simulink model "dblpend1"  (Simulink 6.0)
settings: Solver=ode45  SolverMode=SingleTasking  StartTime=0  StopTime=10000  MaxStep=0.05  RelTol=1e-5  AbsTol=1e-6
PreLoadFcn:
  | l21=5;w21=5;n1=1/4;e1=1/2;
settings Model: Creator=The MathWorks Inc.  LastModifiedBy=batserve  ExtModeTrigMode=oneshot  ExtModeAutoUpdateStatusClock=off
settings DataIOCC: InitialState=xFinal  LimitDataPoints=off  SaveOutput=off  SaveTime=off
settings OptimizationCC: BooleanDataType=off
settings DebuggingCC: CheckExecutionContextPreStartOutputMsg=on  CheckExecutionContextRuntimeOutputMsg=on  SolverPrmCheckMsg=none
settings HardwareCC: TargetUnknown=on

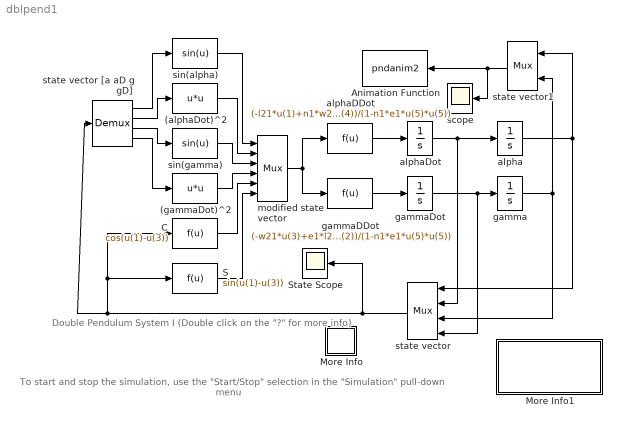
== system dblpend1 ==
  note: Double Pendulum System I
      | (Double click on the "?" for more info)
  note: To start and stop the simulation, use the "Start/Stop"
      | selection in the "Simulation" pull-down menu
  (alphaDot)^2 : Fcn  Expr=u*u
  (gammaDot)^2 : Fcn  Expr=u*u
  Animation Function : S-Function  Orientation=left  FunctionName=pndanim2  Parameters=0.05
      settings: DeleteFcn=if ~isempty(findobj('type','figure','name','dblpend1 Animation'));close('dblpend1 Animation'); end;
  C : Fcn  Expr=cos(u(1)-u(3))
  More Info : Subsystem  PropExecContextAcrossSSBoundary=on
      mask Display: disp('?')
  More Info1 : Subsystem  PropExecContextAcrossSSBoundary=on
      settings: OpenFcn=simcad(bdroot)
      mask Display: disp('Double click\nhere for\nSIMULINK Help')
  S : Fcn  Expr=sin(u(1)-u(3))
  State Scope : Scope
      settings: TickLabels=on  TimeRange=40.000000  YMin=-2.000000  YMax=2.000000  SaveName=ScopeData2  DataFormat=Array
  alpha : Integrator  InitialCondition=100*(pi/180)
  alphaDDot : Fcn  Expr=(-l21*u(1)+n1*w21*u(5)*u(3)-n1*e1*u(5)*u(6)*u(2)-n1*u(6)*u(4))/(1-n1*e1*u(5)*u(5))
  alphaDot : Integrator
  gamma : Integrator  InitialCondition=0*(pi/180)
  gammaDDot : Fcn  Expr=(-w21*u(3)+e1*l21*u(5)*u(1)+n1*e1*u(5)*u(6)*u(4)+e1*u(6)*u(2))/(1-n1*e1*u(5)*u(5))
  gammaDot : Integrator
  modified state vector : Mux  Inputs=6
  scope : Scope
      settings: TickLabels=on  TimeRange=32.000000  YMin=-2.000000  YMax=2.000000  DataFormat=Array
  sin(alpha) : Fcn  Expr=sin(u)
  sin(gamma) : Fcn  Expr=sin(u)
  state vector : Mux  Orientation=left
  state vector [a aD g gD] : Demux
  state vector1 : Mux  Orientation=left  Inputs=2
  wires:
  state vector1/1 -> Animation Function/1, scope/1
  alphaDDot/1 -> alphaDot/1
  gammaDDot/1 -> gammaDot/1
  alphaDot/1 -> alpha/1, state vector/2
  gammaDot/1 -> gamma/1, state vector/4
  alpha/1 -> state vector/1, state vector1/1
  gamma/1 -> state vector/3, state vector1/2
  state vector/1 -> state vector [a aD g gD]/1, C/1, S/1, State Scope/1
  S/1 -> modified state vector/6
  C/1 -> modified state vector/5
  (gammaDot)^2/1 -> modified state vector/4
  sin(gamma)/1 -> modified state vector/3
  (alphaDot)^2/1 -> modified state vector/2
  sin(alpha)/1 -> modified state vector/1
  state vector [a aD g gD]/4 -> (gammaDot)^2/1
  state vector [a aD g gD]/3 -> sin(gamma)/1
  state vector [a aD g gD]/2 -> (alphaDot)^2/1
  state vector [a aD g gD]/1 -> sin(alpha)/1
  modified state vector/1 -> alphaDDot/1, gammaDDot/1

== system dblpend1/More Info ==
  note: This system models a double pendulum system where
      | the rest state has both pendulums hanging vertically.
  note: Associated with the demo is an animation function that
      | will automatically open a figure window and display to it.
  note: Try experimenting with different initial conditions for
      | alpha and gamma to see the unusal coupling effects.

== system dblpend1/More Info1 ==
  note: Try experimenting with different initial conditions for
      | alpha and gamma to see the unusal coupling effects.
  note: Associated with the demo is an animation function that
      | will automatically open a figure window and display to it.
  note: This system models a double pendulum system where
      | the rest state has both pendulums hanging vertically.
